simulink model "quarter_car_suspension"  (R2025b)
settings: Solver=FixedStepAuto  StartTime=0.0  StopTime=10.0  FixedStep=0.01  RelTol=1e-3
undefined symbols (not defined in the file or in its folder): Cs, Ks, Kt, Ms, Mu
libraries: rllib x1
settings Model: Creator=HP  LastModifiedBy=HP

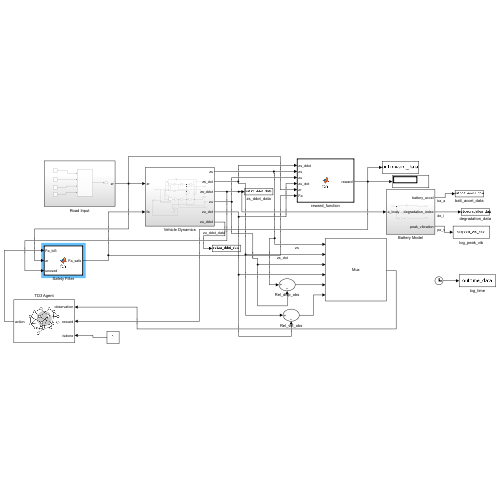
[thumbnail: Simulink's stored preview of the top-level diagram]
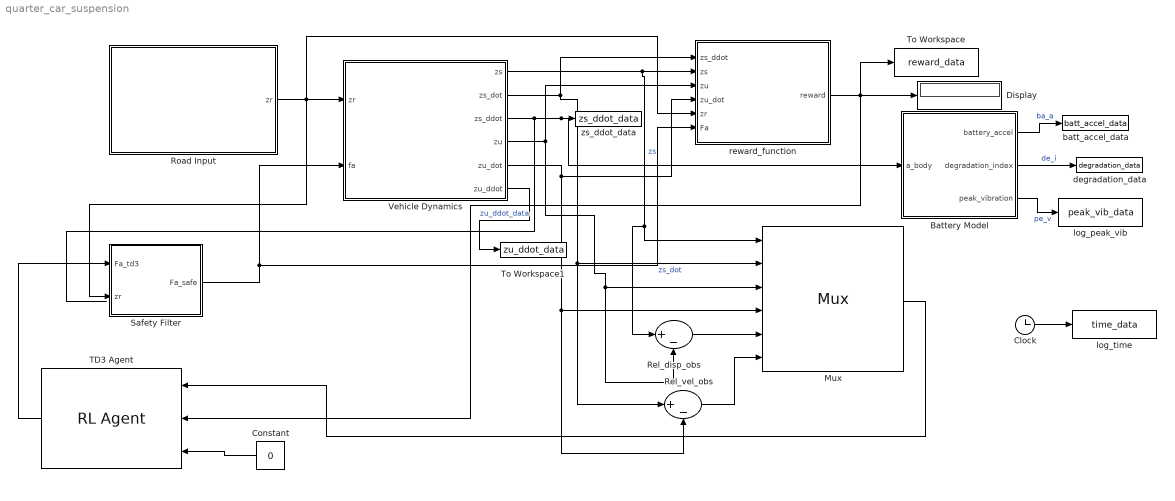
== system quarter_car_suspension ==
  Battery Model : Subsystem
  Clock : Clock
  Constant : Constant  Value=0
  Display : Display
  Mux : Mux  Inputs=6
  Rel_disp_obs : Sum  Inputs=|+-
  Rel_vel_obs : Sum  Inputs=|+-
  Road Input : Subsystem
  Safety Filter : MATLAB Function  TreatAsAtomicUnit=on
  TD3 Agent : rllib/RL Agent  Agent=agentObj  ExternalActionAsInput=off  ProvideLastAction=off  ProvideCumRwd=off  TreatAsDirectFeedthrough=on  UseStrictObservationDataTypes=off
  To Workspace : ToWorkspace  VariableName=reward_data  SaveFormat=Timeseries  SampleTime=-1
  To Workspace1 : ToWorkspace  VariableName=zu_ddot_data  SampleTime=-1
  Vehicle Dynamics : Subsystem
  batt_accel_data : ToWorkspace  VariableName=batt_accel_data  SampleTime=-1
  degradation_data : ToWorkspace  VariableName=degradation_data  SampleTime=-1
  log_peak_vib : ToWorkspace  VariableName=peak_vib_data  SampleTime=-1
  log_time : ToWorkspace  VariableName=time_data  SampleTime=-1
  reward_function : MATLAB Function  TreatAsAtomicUnit=on
  zs_ddot_data : ToWorkspace  VariableName=zs_ddot_data  SampleTime=-1
  wires:
  Road Input/1(zr) -> Safety Filter/2(zr), reward_function/5(zr), Vehicle Dynamics/1(zr)
  Vehicle Dynamics/3(zs_ddot) -> zs_ddot_data/1, Battery Model/1(a_body)
  Vehicle Dynamics/1(zs) -> reward_function/2(zs), Mux/1, Rel_disp_obs/1  "zs"
  Vehicle Dynamics/2(zs_dot) -> reward_function/1(zs_ddot), Rel_vel_obs/1, Mux/2  "zs_dot"
  Vehicle Dynamics/4(zu) -> reward_function/3(zu), Rel_disp_obs/2, Mux/3
  Vehicle Dynamics/5(zu_dot) -> reward_function/4(zu_dot), Rel_vel_obs/2, Mux/4
  Rel_disp_obs/1 -> Mux/5
  Rel_vel_obs/1 -> Mux/6
  Mux/1 -> TD3 Agent/1
  reward_function/1(reward) -> Display/1, To Workspace/1, TD3 Agent/2
  Constant/1 -> TD3 Agent/3
  Vehicle Dynamics/6(zu_ddot) -> To Workspace1/1  "zu_ddot_data"
  Battery Model/1(battery_accel) -> batt_accel_data/1  "ba_a"
  Battery Model/2(degradation_index) -> degradation_data/1  "de_i"
  Battery Model/3(peak_vibration) -> log_peak_vib/1  "pe_v"
  Clock/1 -> log_time/1
  TD3 Agent/1 -> Safety Filter/1(Fa_td3)
  Safety Filter/1(Fa_safe) -> reward_function/6(Fa), Vehicle Dynamics/2(fa)

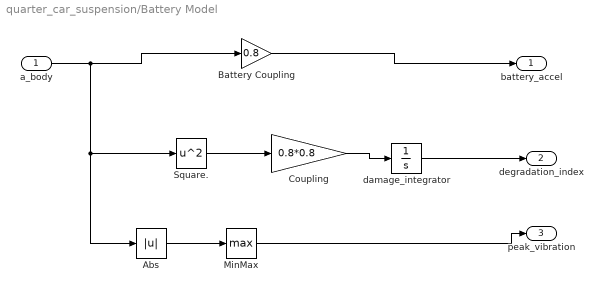
== system quarter_car_suspension/Battery Model ==
  a_body : Inport
  Abs : Abs  SaturateOnIntegerOverflow=off
  Battery Coupling : Gain  Gain=0.8
  Coupling : Gain  Gain=0.8*0.8
  MinMax : MinMax  Function=max
  Square. : Math  Operator=square
  damage_integrator : Integrator
  battery_accel : Outport
  degradation_index : Outport  Port=2
  peak_vibration : Outport  Port=3
  wires:
  a_body/1 -> Abs/1, Square./1, Battery Coupling/1
  Battery Coupling/1 -> battery_accel/1
  Square./1 -> Coupling/1
  Coupling/1 -> damage_integrator/1
  damage_integrator/1 -> degradation_index/1
  Abs/1 -> MinMax/1
  MinMax/1 -> peak_vibration/1

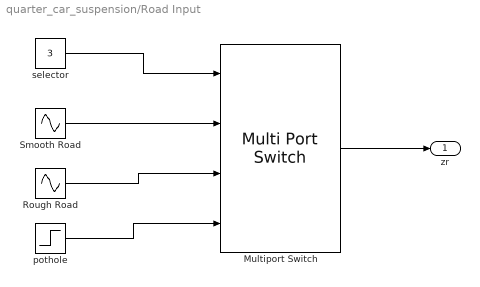
== system quarter_car_suspension/Road Input ==
  Multiport Switch : MultiPortSwitch  SaturateOnIntegerOverflow=off  InputSameDT=off
  Rough Road : Sin  Amplitude=0.02  Frequency=5  SampleTime=0
  Smooth Road : Sin  Amplitude=0.01  Frequency=2  SampleTime=0
  pothole : Step  After=0.03  SampleTime=0
  selector : Constant  Value=3
  zr : Outport
  wires:
  selector/1 -> Multiport Switch/1
  Smooth Road/1 -> Multiport Switch/2
  Rough Road/1 -> Multiport Switch/3
  pothole/1 -> Multiport Switch/4
  Multiport Switch/1 -> zr/1

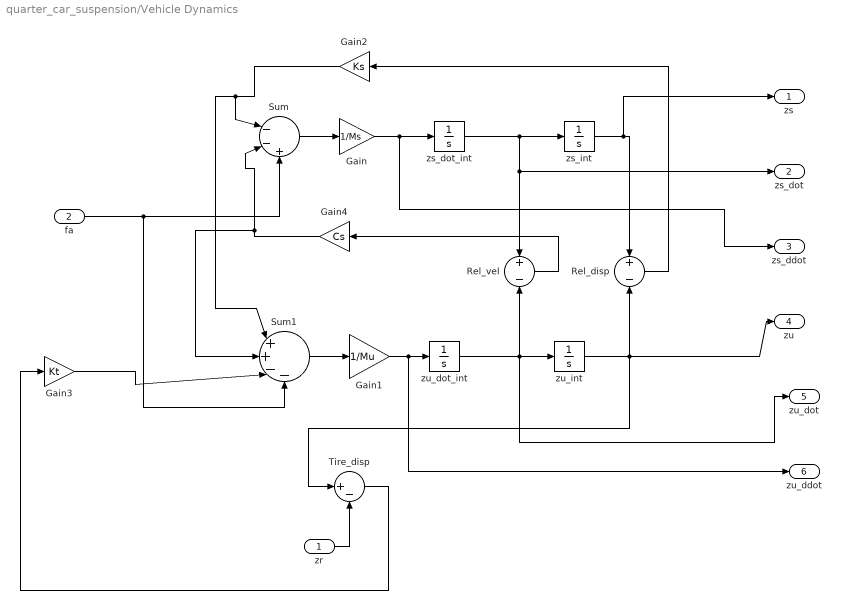
== system quarter_car_suspension/Vehicle Dynamics ==
  zr : Inport
  fa : Inport  Port=2
  Gain : Gain  Gain=1/Ms
  Gain1 : Gain  Gain=1/Mu
  Gain2 : Gain  Gain=Ks
  Gain3 : Gain  Gain=Kt
  Gain4 : Gain  Gain=Cs
  Rel_disp : Sum  Inputs=+|-
  Rel_vel : Sum  Inputs=+|-
  Sum : Sum  Inputs=|--+
  Sum1 : Sum  Inputs=|++--
  Tire_disp : Sum  Inputs=|+-
  zs_dot_int : Integrator
  zs_int : Integrator
  zu_dot_int : Integrator
  zu_int : Integrator
  zs : Outport
  zs_dot : Outport  Port=2
  zs_ddot : Outport  Port=3
  zu : Outport  Port=4
  zu_dot : Outport  Port=5
  zu_ddot : Outport  Port=6
  wires:
  Sum/1 -> Gain/1
  Gain/1 -> zs_ddot/1, zs_dot_int/1
  zs_dot_int/1 -> zs_dot/1, Rel_vel/1, zs_int/1
  Gain1/1 -> zu_ddot/1, zu_dot_int/1
  zu_dot_int/1 -> zu_dot/1, Rel_vel/2, zu_int/1
  Sum1/1 -> Gain1/1
  zs_int/1 -> zs/1, Rel_disp/1
  zu_int/1 -> Rel_disp/2, zu/1, Tire_disp/1
  Rel_disp/1 -> Gain2/1
  Gain2/1 -> Sum/1, Sum1/1
  Rel_vel/1 -> Gain4/1
  Gain4/1 -> Sum1/2, Sum/2
  zr/1 -> Tire_disp/2
  fa/1 -> Sum/3, Sum1/4
  Gain3/1 -> Sum1/3
  Tire_disp/1 -> Gain3/1

== matlab function quarter_car_suspension/Safety Filter ==
  data: Fa_td3 input; Fa_safe output; zr input
function Fa_safe = fcn(Fa_td3, zr)

pothole_detected = abs(zr) > 0.02;

if pothole_detected
  
    Fa_safe = 0.0;
else
    % Full TD3 control on smooth/rough roads
    Fa_safe = Fa_td3;
end
end

== matlab function quarter_car_suspension/reward_function ==
  data: zs_ddot input; reward output; zs input; zu input; zu_dot input; zr input; Fa input
function reward = fcn(zs_ddot, zs, zu, zu_dot, zr, Fa)
%#codegen
accel_g   = zs_ddot / 9.81;
batt_g    = (0.8 * zs_ddot) / 9.81;
susp_defl = zs - zu;
tire_defl = zu - zr;
event_mag = abs(zs_ddot);
alpha = 1.0 / (1.0 + exp(-1.2 * (event_mag - 3.0)));
w_comfort = 0.65 - 0.35 * alpha;
w_battery = 0.20 + 0.35 * alpha;
comfort_term  = -3.0 * accel_g * accel_g;
battery_term  = -3.0 * batt_g  * batt_g;
comfort_bonus = 0.0;
battery_bonus = 0.0;
susp_norm = susp_defl / 0.08;
if abs(susp_norm) >= 1.0
    stability_penalty = 1.0 + 1.5 * (abs(susp_norm) - 1.0);
else
    stability_penalty = susp_norm * susp_norm;
end
tire_norm = tire_defl / 0.04;
if abs(tire_norm) >= 1.0
    road_penalty = 1.0;
else
    road_penalty = tire_norm * tire_norm;
end
effort_penalty = 0.02 * (Fa / 5000.0) * (Fa / 5000.0);
if abs(accel_g) > 2.0
    large_accel_penalty = 2.0 * (abs(accel_g) - 2.0)^2;
else
    large_accel_penalty = 0.0;
end
reward = w_comfort * (comfort_term + comfort_bonus)
       + w_battery * (battery_term + battery_bonus)
       - 0.10 * stability_penalty
       - 0.05 * road_penalty
       - 0.01 * zu_dot * zu_dot
       - effort_penalty
       - large_accel_penalty;
if reward < -5.0
    reward = -5.0;
end
end
